simulink model "gtm_design"  (R2025b)
settings: Solver=ode2  StartTime=0.0  StopTime=1000  FixedStep=Timestep  MaxStep=0.1  MinStep=0.005  RelTol=1e-5
StopFcn:
  | MWSout=grabmws(bdroot);
  | MWSout.lastrun=datestr(now);
values from neighbouring files (symbols this model uses):
  AltMap = [0 20 40 60 80 100 120 140 160 180 200 220 ... (2938 elements, 1469x2)]    [WPs.mat]    (also in create_WPs.m = [s_alt, alt_ref])
  ApproachParams = [29.3870633886 40.9266984885 1000 29.3345096172 40.9077524395 408.9474942 29.321008 40.902885 318.9474942 244.5 2.5 90]    [WPs.mat]    (also in alternative_trajectory.mat; create_WPs.m = TRJ.ApproachParams; guidance.m = [; trajectory.mat)
  psi_deg = [0 0 0 0 0 0 0 0 0 0 0 0 ... (60 elements, 60x1)]    [WPs.mat]    (also in create_WPs.m = zeros(size(lat_wp)))
  WPs = [29.3 29.3 29.3 29.3 29.3 29.3 29.3 29.3 29.3 29.3 29.3 29.3 ... (240 elements, 60x4)]    [WPs.mat]    (also in create_WPs.m = [      lon_wp,      lat_wp,      alt_wp,      tas_kts])
undefined symbols (not defined in the file or in its folder): Aero, aftfuel, aftfuel_pos, AILL, AILLC, AILR, AILRC, alpha_deg, altitude_ft, Ax_g, Ay_g, Az_g, b, beta_deg, bias, BRAKEC, Cbar, cg_pos0, cg_shift_gear, DamageCase, DamageModels, DamageOnsetTime, ELLIB, ELLIBC, ELLOB, ELLOBC, ELRIB, ELRIBC, ELROB, ELROBC, engl_ang, engl_pos, engr_ang, engr_pos, FLAPLIB, FLAPLIC, FLAPLOB, FLAPLOC, FLAPRIB, FLAPRIC, FLAPROB, FLAPROC, FuelUsed_Init, fwdfuel, fwdfuel_pos, GEAR, GEARC, Inertia0, Inertia_shift_gear, InitialTime, Ixx_model, Iyy_model, Izz_model, KTAS, LandingGear, LengON, LinearizeModeOn, ln, NAV_altitude_m, NAV_latitude_deg ... (+62)
libraries: simulink_need_slupdate x30, simulink x11, slpidlib x7, simulink_extras x6, aerolibfltsims x2
(part 8 of 8)

== system gtm_design/Input Generator/Winds/Turbulence  Model/Dryden Model/Longitudinal Turbulence/filter parameters/Tm-4511 severe data ==
  note: "Light" and "Moderate" sigmas are ZERO below 1km alt.
      | Table 2-79 does not define them.
  "alt, m" : Inport
  intensity : Inport  Port=2
  "Longitudinal Scale, m TM-4511 Table 2-79" : Lookup  InputValues=[0 10 20 30 40 50 60 70 80 90 100 200 304.8 305 762 769 900 1000 2000 4000 6000 8000 10000 12000 14000 16000]  Table=[21 21 33 43 52 61 68 75 82 89 95 149 196 300 300 533 533 832 902 1040 1040 1040 1230 1800 2820 3400]
  "Longitudinal sigma, m/s light TM-4511 Table 2-79" : Lookup  InputValues="[10 20 30 40 50 60 70 80 90 100 200 304.8 305 400  762 769 1000 2000 4000 6000 8000 10000 12000 14000 16000]"  Table="[0   0   0   0   0   0   0   0   0    0    0    0   0   0   0   0   .17  .17  .2   .21   .22   .22   .25   .26   .24   ]"
  "Longitudinal sigma, m/s moderate TM-4511 Table 2-79" : Lookup  InputValues="[10 20 30 40 50 60 70 80 90 100 200 304.8 305 400  762 769 1000 2000 4000 6000 8000 10000 12000 14000 16000]"  Table="[0   0  0    0    0   0  0  0   0   0     0    0      0     0      0    0  1.65  1.65 2.04 2.13 2.15 2.23 2.47 2.62 2.44]"
  "Longitudinal sigma, m/s severe TM-4511 Table 2-79" : Lookup  InputValues="[10 20 30 40 50 60 70 80 90 100 200 304.8 305 400  762 769 1000 2000 4000 6000 8000 10000 12000 14000 16000]"  Table=[2.31 2.58 2.75 2.88 2.98 3.07 3.15 3.22 3.28 3.33 3.72 3.95 4.37 4.39 4.39 5.7 5.7 5.8 6.24 7.16 7.59 7.72 7.89 6.93 5]
  Multiport Switch : MultiPortSwitch
  "sigma, m/s" : Outport
  "scale length, m" : Outport  Port=2
  wires:
  "alt, m"/1 -> "Longitudinal sigma, m/s severe TM-4511 Table 2-79"/1, "Longitudinal Scale, m TM-4511 Table 2-79"/1, "Longitudinal sigma, m/s moderate TM-4511 Table 2-79"/1, "Longitudinal sigma, m/s light TM-4511 Table 2-79"/1
  "Longitudinal Scale, m TM-4511 Table 2-79"/1 -> "scale length, m"/1
  Multiport Switch/1 -> "sigma, m/s"/1
  "Longitudinal sigma, m/s severe TM-4511 Table 2-79"/1 -> Multiport Switch/4
  "Longitudinal sigma, m/s moderate TM-4511 Table 2-79"/1 -> Multiport Switch/3
  "Longitudinal sigma, m/s light TM-4511 Table 2-79"/1 -> Multiport Switch/2
  intensity/1 -> Multiport Switch/1

== system gtm_design/Input Generator/Winds/Turbulence  Model/Dryden Model/Vertical Turbulence/SubSystem/MIL-STD-1797A APPENDIX A  ==
  note: This data from Fig 262, pg 652
  "alt, m" : Inport
  intensity : Inport  Port=2
  "0.1*mean wind, fps sigma w = to 2.5f/s * intensity Fig 263, pg 654" : Gain  Gain=2.5  SaturateOnIntegerOverflow=on  OutDataTypeStr=Inherit: Same as input  ParamDataTypeStr=Inherit: Same as input
  1 : Constant  Value=500
  2 : Constant  Value=.15
  Demux : Demux  Outputs=2
      settings: DisplayOption=none
  "L w = min(500, alt/2)" : Fcn  Expr=u(1)/2
  "Light sigma, f/s" : Lookup  InputValues=[2000 9000 18000 100000]  Table=[5 5 3 3]
  MinMax : MinMax  Inputs=2  InputSameDT=on  SaturateOnIntegerOverflow=on
  MinMax1 : MinMax  Function=max  Inputs=2  InputSameDT=on  SaturateOnIntegerOverflow=on
  Multiport Switch : MultiPortSwitch
  Mux : Mux  Inputs=2
  Mux1 : Mux  Inputs=2
  Product : Product  InputSameDT=on  SaturateOnIntegerOverflow=on  OutDataTypeStr=Inherit: Same as first input
  "Scale Length, ft" : Constant  Value=1750/2
  Ux / U20 : Fcn  Expr=ln(u(1)/.15)/ln(20/.15)
  alt >2000 ft : Switch  Threshold=2000
  "ft -> m" : Gain  Gain=.3048  SaturateOnIntegerOverflow=on  OutDataTypeStr=Inherit: Same as input  ParamDataTypeStr=Inherit: Same as input
  "m -> ft" : Gain  Gain=1/.3048  SaturateOnIntegerOverflow=on  OutDataTypeStr=Inherit: Same as input  ParamDataTypeStr=Inherit: Same as input
  "moderate sigma, f/s" : Lookup  InputValues=[2000 12000 44000 100000]  Table=[10 10 3 3]
  "severe sigma, f/s" : Lookup  InputValues=[2000 5000 22000 80000 100000]  Table=[15.5 21.5 21.5 3 3]
  "sigma, m/s" : Outport
  "scale length, m" : Outport  Port=2
  wires:
  "Light sigma, f/s"/1 -> Multiport Switch/2
  "moderate sigma, f/s"/1 -> Multiport Switch/3
  "severe sigma, f/s"/1 -> Multiport Switch/4
  "alt, m"/1 -> "m -> ft"/1
  Multiport Switch/1 -> Mux/1
  Mux/1 -> alt >2000 ft/1
  intensity/1 -> Multiport Switch/1, "0.1*mean wind, fps sigma w = to 2.5f/s * intensity Fig 263, pg 654"/1
  "Scale Length, ft"/1 -> Mux/2
  "m -> ft"/1 -> alt >2000 ft/2, "severe sigma, f/s"/1, "Light sigma, f/s"/1, "moderate sigma, f/s"/1, "L w = min(500, alt/2)"/1, MinMax1/2
  Mux1/1 -> alt >2000 ft/3
  Demux/2 -> "scale length, m"/1
  Demux/1 -> "sigma, m/s"/1
  alt >2000 ft/1 -> "ft -> m"/1
  "ft -> m"/1 -> Demux/1
  1/1 -> MinMax/1
  "L w = min(500, alt/2)"/1 -> MinMax/2
  2/1 -> MinMax1/1
  MinMax1/1 -> Ux / U20/1
  Ux / U20/1 -> Product/2
  "0.1*mean wind, fps sigma w = to 2.5f/s * intensity Fig 263, pg 654"/1 -> Product/1
  Product/1 -> Mux1/1
  MinMax/1 -> Mux1/2

== system gtm_design/Input Generator/Winds/Turbulence  Model/Dryden Model/Vertical Turbulence/SubSystem/Tm-4511 severe data ==
  note: "Light" and "Moderate" sigmas are ZERO below 1km alt.
      | Table 2-79 does not define them.
  "alt, m" : Inport
  intensity : Inport  Port=2
  Multiport Switch : MultiPortSwitch
  "Vertical sigma, m/s light TM-4511 Table 2-79" : Lookup  InputValues="[10 20 30 40 50 60 70 80 90 100 200 304.8 305 400  762 769 1000 2000 4000 6000 8000 10000 12000 14000 16000]"  Table="[0   0   0   0   0   0   0   0   0    0    0    0   0   0   0   0   .14  .14  .17   .17   .17   .17   .18   .19   .21   ]"
  "Vertical sigma, m/s moderate TM-4511 Table 2-79" : Lookup  InputValues="[10 20 30 40 50 60 70 80 90 100 200 304.8 305 400  762 769 1000 2000 4000 6000 8000 10000 12000 14000 16000]"  Table="[0   0  0    0    0   0  0  0   0   0     0    0      0     0      0    0  1.36  1.43 1.68 1.69 1.695 1.73 1.79 1.91 2.1]"
  "Vertical Scale, m TM-4511 Table 2-79" : Lookup  InputValues=[0 10 20 30 40 50 60 70 80 90 100 200 304.8 305 762 769 900 1000 2000 4000 6000 8000 10000 12000 14000 16000]  Table=[ 5 5 11 17 23 29 35 41 47 53 59 123 192 300 300 533 533 624 831 972 1010 980 1100 1540 2120 2600]
  "Vertical sigma, m/s severe TM-4511 Table 2-79" : Lookup  InputValues=[10 20 30 40 50 60 70 80 90 100 200 304.8 305 762 769 900 1000 2000 4000 6000 8000 10000 12000 14000 16000]  Table=[1.15 1.46 1.71 1.89 2.05 2.19 2.32 2.43 2.54 2.64 3.38 3.95 4.39 4.39 5.7 5.7 4.67 4.75 5.13 5.69 5.98 6 5.71 5.05 4.31]
  "sigma, m/s" : Outport
  "scale length, m" : Outport  Port=2
  wires:
  "alt, m"/1 -> "Vertical Scale, m TM-4511 Table 2-79"/1, "Vertical sigma, m/s severe TM-4511 Table 2-79"/1, "Vertical sigma, m/s moderate TM-4511 Table 2-79"/1, "Vertical sigma, m/s light TM-4511 Table 2-79"/1
  "Vertical Scale, m TM-4511 Table 2-79"/1 -> "scale length, m"/1
  Multiport Switch/1 -> "sigma, m/s"/1
  "Vertical sigma, m/s moderate TM-4511 Table 2-79"/1 -> Multiport Switch/3
  "Vertical sigma, m/s light TM-4511 Table 2-79"/1 -> Multiport Switch/2
  intensity/1 -> Multiport Switch/1
  "Vertical sigma, m/s severe TM-4511 Table 2-79"/1 -> Multiport Switch/4

== matlab function gtm_design/GTM_T2/EOM/Aircraft 6DOF/EulerDot ==
  data: pqr input size=3; deuler output size=3; euler input size=3
function deuler = e2de(pqr,euler)
% This block supports an embeddable subset of the MATLAB language.
% See the help menu for details. 

P=pqr(1);
Q=pqr(2);
R=pqr(3);

phi=euler(1);
theta=euler(2);
psi=euler(3);

c_phi=cos(phi);
s_phi=sin(phi);
c_theta=cos(theta);
s_theta=sin(theta);

phi_dot   = P + (1/c_theta)*(s_phi*s_theta*Q + c_phi*s_theta*R);
theta_dot = c_phi*Q - s_phi*R;
psi_dot   = (1/c_theta)*(s_phi*Q + c_phi*R);

deuler=[phi_dot; theta_dot; psi_dot];

== matlab function gtm_design/GTM_T2/EOM/Aircraft 6DOF/Form Inertia Matrix ==
  data: Ixx input double size=1; I output size=[3 3]; Iyy input size=1; Izz input size=1; Ixz input size=1; Iyz input size=1; Ixy input size=1; InvI output size=[3 3]
function [I,InvI] = Inertia(Ixx,Iyy,Izz,Ixz,Iyz,Ixy)
% This block supports an embeddable subset of the MATLAB language.
% See the help menu for details. 

I=[ Ixx, -Ixy, -Ixz;
   -Ixy,  Iyy, -Iyz;
   -Ixz, -Iyz,   Izz ];

det = Ixx*Iyy*Izz-Ixx*Iyz^2-Ixy^2*Izz-2*Ixy*Ixz*Iyz-Ixz^2*Iyy;

adjoint=[...
Iyy*Izz-Iyz^2,    Ixy*Izz+Ixz*Iyz, Ixy*Iyz+Ixz*Iyy;...
Ixy*Izz+Ixz*Iyz,   Ixx*Izz-Ixz^2,  Ixx*Iyz+Ixy*Ixz;...
Ixy*Iyz+Ixz*Iyy,  Ixx*Iyz+Ixy*Ixz,   Ixx*Iyy-Ixy^2     ];

InvI=adjoint/det;

== matlab function gtm_design/GTM_T2/Engines/Engine Alignment ==
  data: T output; Tl input; hl input; Tr input; hr input; TL output; engl_ang parameter; engr_ang parameter; TR output; H output
function [T,TL,TR,H] = eng_angles(Tl,hl,Tr,hr,engl_ang,engr_ang)
% This block supports an embeddable subset of the MATLAB language.
% See the help menu for details. 

% Using the engine alignment angles (set in AC_params_T2.m), compute the 
% off-axis thrust and angular momentum terms.

TL = Tl*[cosd(engl_ang(2))*cosd(engl_ang(3));...
         sind(engl_ang(3));...
         -sind(engl_ang(2))*cosd(engl_ang(3))];
TR = Tr*[cosd(engr_ang(2))*cosd(engr_ang(3));...
         sind(engr_ang(3));...
         -sind(engr_ang(2))*cosd(engr_ang(3))];  
T = TL+TR;

H = hl*[cosd(engl_ang(2))*cosd(engl_ang(3));...
         sind(engl_ang(3));...
         -sind(engl_ang(2))*cosd(engl_ang(3))] + ...
         hr*[cosd(engr_ang(2))*cosd(engr_ang(3));...
         sind(engr_ang(3));...
         -sind(engr_ang(2))*cosd(engr_ang(3))];

== matlab function gtm_design/GTM_T2/Engines/Left_Engine Jetcat P70/Simple Ram Drag Model ==
  data: ram_drag output; qbar input; S input; ram_drag_coef parameter
function ram_drag =   ram_drag(qbar,S,ram_drag_coef)
% This block supports the Embedded MATLAB subset.
% See the help menu for details. 

ram_drag = ram_drag_coef.*qbar.*S;
return

== matlab function gtm_design/GTM_T2/Engines/Right_Engine Jetcat P70/Simple Ram Drag Model ==
  data: ram_drag output; qbar input; S input; ram_drag_coef parameter
function ram_drag =   ram_drag(qbar,S,ram_drag_coef)
% This block supports the Embedded MATLAB subset.
% See the help menu for details. 

ram_drag = ram_drag_coef.*qbar.*S;
return

== matlab function gtm_design/Input Generator/FCS/Waypoint Tracking ==
  settings: updateMethod=DISCRETE  sampleTime=0.01
  data: lon_deg input; h_ref output; lat_deg input; alt_ft input; psi_deg input; TAS_kts input; beta_deg input; WPs input; AltMap input; ApproachParams input; Ts input; reset input; psi_ref output; TAS_ref output; beta_ref output; wp_idx output; status output; e_ct output; dist_to_wp output; along_m output
function [h_ref, psi_ref, TAS_ref, beta_ref, wp_idx, status, e_ct, dist_to_wp, along_m] = ...
    WP_Tracker(lon_deg, lat_deg, alt_ft, psi_deg, TAS_kts, beta_deg, WPs, AltMap, ApproachParams, Ts, reset)
%#codegen
%
% WPs format:
%   WPs(:,1) = lon_deg
%   WPs(:,2) = lat_deg
%   WPs(:,3) = alt_ft
%   WPs(:,4) = TAS_kts
%
% AltMap format:
%   AltMap(:,1) = station_m
%   AltMap(:,2) = alt_ref_ft
%
% ApproachParams format:
%   1  = FAF_lon_deg
%   2  = FAF_lat_deg
%   3  = FAF_alt_ft
%   4  = FLARE_lon_deg
%   5  = FLARE_lat_deg
%   6  = FLARE_alt_ft
%   7  = TD_lon_deg
%   8  = TD_lat_deg
%   9  = TD_alt_ft
%   10 = runway_heading_deg
%   11 = glide_angle_deg
%   12 = flare_alt_agl_ft

%% ============================================================
% USER PARAMETERS
% =============================================================

lat0_deg = 40.88;
lon0_deg = 29.30;

% Normal WP acceptance
R_accept_m = 80.0;

% Turn WP acceptance
% Dönüş waypointlerinde daha erken segment değişimi için kullanılır.
% 220-300 m arası denenebilir.
R_accept_turn_m = 320.0;

% Bir WP'nin dönüş WP'si sayılması için minimum rota değişimi
turn_angle_min_deg = 25.0;

R_final_m = 50.0;

lookahead_time_s = 4.0;
Ld_min_m = 80.0;
Ld_max_m = 450.0;

psi_exp_small_err_deg = 25.0;
psi_exp_large_err_deg = 65.0;

chi_corr_lim_deg = 30.0;

exp_Ld_factor = 1.5;
exp_Ld_min_m  = 150.0;
exp_Ld_max_m  = 800.0;

psi_rate_lim_degps = 20.0;
h_rate_lim_ftps    = 25.0;
TAS_rate_lim_ktsps = 5.0;

TAS_min_kts = 0.0;
TAS_max_kts = 120.0;

% Normal AltMap station protection
alt_back_window_m = 30.0;
alt_fwd_window_min_m = 150.0;
alt_fwd_window_time_s = 5.0;
alt_station_rate_gain = 1.10;

% Approach geometry activation gates
approach_pre_faf_margin_m = 1500.0;
approach_xtrack_gate_m    = 1200.0;
approach_after_td_m       = 500.0;

% Smooth vertical curve at FAF
faf_vertical_curve_m = 600.0;

%% ============================================================
% PERSISTENT STATES
% =============================================================

persistent targetIdx initialized ...
           startN startE startAlt startTAS ...
           hLast psiLast TASLast ...
           sAltLast

if isempty(initialized) || reset > 0.5

    targetIdx = int32(1);

    [startN, startE] = ll2ne_simple(lat_deg, lon_deg, lat0_deg, lon0_deg);

    startAlt = alt_ft;
    startTAS = TAS_kts;

    hLast   = alt_ft;
    psiLast = wrap180(psi_deg);
    TASLast = TAS_kts;

    sAltLast = 0.0;

    initialized = true;

end

Ts_eff = max(Ts, 1.0e-6);

Nwp = int32(size(WPs, 1));

%% ============================================================
% EMPTY / INVALID MISSION PROTECTION
% =============================================================

if Nwp < int32(1)

    h_ref      = alt_ft;
    psi_ref    = wrap180(psi_deg);
    TAS_ref    = TAS_kts;
    beta_ref   = 0.0;
    wp_idx     = 0.0;
    status     = -1.0;
    e_ct       = 0.0;
    dist_to_wp = 0.0;
    along_m    = 0.0;

    return;

end

if targetIdx < int32(1)
    targetIdx = int32(1);
end

if targetIdx > Nwp
    targetIdx = Nwp;
end

%% ============================================================
% CURRENT AIRCRAFT POSITION IN LOCAL NORTH-EAST FRAME
% =============================================================

[pN, pE] = ll2ne_simple(lat_deg, lon_deg, lat0_deg, lon0_deg);

%% ============================================================
% ADVANCE WAYPOINT IF NEEDED
% =============================================================

for iter = 1:200

    if iter > double(Nwp)
        break;
    end

    [AN, AE, ~, ~] = getSegmentStart(targetIdx, WPs, ...
        startN, startE, startAlt, startTAS, lat0_deg, lon0_deg);

    [BN, BE, ~, ~] = getWaypoint(targetIdx, WPs, lat0_deg, lon0_deg);

    dN = BN - AN;
    dE = BE - AE;

    L = sqrt(dN*dN + dE*dE);

    if L < 1.0

        qN = cosd(psiLast);
        qE = sind(psiLast);
        s  = 0.0;

    else

        qN = dN / L;
        qE = dE / L;
        s  = (pN - AN)*qN + (pE - AE)*qE;

    end

    dToB_N = pN - BN;
    dToB_E = pE - BE;
    distB  = sqrt(dToB_N*dToB_N + dToB_E*dToB_E);

    e_ct_switch = -qE*(pN - AN) + qN*(pE - AE);

    % ------------------------------------------------------------
    % Turn-aware waypoint acceptance radius
    % ------------------------------------------------------------
    % Düz WP'lerde normal radius kullanılır.
    % Dönüş WP'lerinde daha büyük radius kullanılır.
    %
    % Bu sayede tracker dönüş WP'sine çok geç kalmadan bir sonraki
    % segmente geçer ve psi_ref köşeli kırılmak yerine daha erken
    % dönmeye başlar.

    isTurnWP = isTurningWaypoint(targetIdx, WPs, startN, startE, ...
        lat0_deg, lon0_deg, turn_angle_min_deg);

    if isTurnWP
        R_accept_eff = R_accept_turn_m;
    else
        R_accept_eff = R_accept_m;
    end

    passed_halfplane = (s >= L);
    near_wp = (distB <= R_accept_eff);
    near_path_lateral = (abs(e_ct_switch) <= R_accept_eff);

    if targetIdx < Nwp && (near_wp || (passed_halfplane && near_path_lateral) || L < 1.0)
        targetIdx = targetIdx + int32(1);
    else
        break;
    end

end

%% ============================================================
% ACTIVE SEGMENT GEOMETRY
% =============================================================

[AN, AE, Aalt, ATAS] = getSegmentStart(targetIdx, WPs, ...
    startN, startE, startAlt, startTAS, lat0_deg, lon0_deg);

[BN, BE, Balt, BTAS] = getWaypoint(targetIdx, WPs, lat0_deg, lon0_deg);

dN = BN - AN;
dE = BE - AE;

L = sqrt(dN*dN + dE*dE);

if L < 1.0

    qN = cosd(psiLast);
    qE = sind(psiLast);
    s  = 0.0;

else

    qN = dN / L;
    qE = dE / L;
    s  = (pN - AN)*qN + (pE - AE)*qE;

end

s_clamped = sat(s, 0.0, max(L, 1.0));

e_ct = -qE*(pN - AN) + qN*(pE - AE);

dToB_N = pN - BN;
dToB_E = pE - BE;
dist_to_wp = sqrt(dToB_N*dToB_N + dToB_E*dToB_E);

along_m = s;

%% ============================================================
% LOOKAHEAD / CARROT POINT
% =============================================================

TAS_ms = max(TAS_kts, 1.0) * 0.514444;

Ld = lookahead_time_s * TAS_ms;
Ld = sat(Ld, Ld_min_m, Ld_max_m);

if L < 1.0
    s_LA = 0.0;
else
    s_LA = sat(s_clamped + Ld, 0.0, L);
end

alpha_LA = 1.0;

if L >= 1.0
    alpha_LA = sat(s_LA / L, 0.0, 1.0);
end

N_LA = AN + alpha_LA*dN;
E_LA = AE + alpha_LA*dE;

dLA_N = N_LA - pN;
dLA_E = E_LA - pE;

dist_LA = sqrt(dLA_N*dLA_N + dLA_E*dLA_E);

if dist_LA < 1.0
    psi_carrot = psiLast;
else
    psi_carrot = atan2d(dLA_E, dLA_N);
end

psi_carrot = wrap180(psi_carrot);

%% ============================================================
% HYBRID PSI REFERENCE GENERATION
% =============================================================

psi_carrot_raw = psi_carrot;

if L < 1.0
    chi_path = psiLast;
else
    chi_path = atan2d(qE, qN);
end

chi_path = wrap180(chi_path);

Ld_exp = exp_Ld_factor * Ld;
Ld_exp = sat(Ld_exp, exp_Ld_min_m, exp_Ld_max_m);

chi_corr = atan2d(-e_ct, Ld_exp);
chi_corr = sat(chi_corr, -chi_corr_lim_deg, chi_corr_lim_deg);

psi_exp_raw = wrap180(chi_path + chi_corr);

err_heading_path   = abs(wrap180(chi_path       - psi_deg));
err_heading_carrot = abs(wrap180(psi_carrot_raw - psi_deg));

heading_err_for_mode = min(err_heading_path, err_heading_carrot);

blend_den = max(psi_exp_large_err_deg - psi_exp_small_err_deg, 1.0);

mu_carrot = (heading_err_for_mode - psi_exp_small_err_deg) / blend_den;
mu_carrot = smoothstep01(mu_carrot);

psi_raw = angleLerpDeg(psi_exp_raw, psi_carrot_raw, mu_carrot);

if heading_err_for_mode < psi_exp_small_err_deg
    psi_raw = psi_exp_raw;
end

psi_raw = wrap180(psi_raw);

%% ============================================================
% ALTITUDE AND TAS REFERENCES
% =============================================================

% ------------------------------------------------------------
% 1) Normal altitude from AltMap
% ------------------------------------------------------------

alt_fwd_window_m = max(alt_fwd_window_min_m, TAS_ms * alt_fwd_window_time_s);

s_alt_candidate = getMissionStationClosestWindowed( ...
    pN, pE, WPs, startN, startE, lat0_deg, lon0_deg, ...
    sAltLast, alt_back_window_m, alt_fwd_window_m);

if s_alt_candidate < sAltLast
    s_alt_candidate = sAltLast;
end

sAlt_rate_max = max(TAS_ms, 1.0) * alt_station_rate_gain;
sAlt_step_max = sAlt_rate_max * Ts_eff;

if s_alt_candidate > sAltLast + sAlt_step_max
    s_alt = sAltLast + sAlt_step_max;
else
    s_alt = s_alt_candidate;
end

sAltLast = s_alt;

h_fallback = Aalt + alpha_LA*(Balt - Aalt);
h_altmap = getAltFromMap(s_alt, AltMap, h_fallback);

% ------------------------------------------------------------
% 2) Approach altitude protection / override
% ------------------------------------------------------------
%
% appMode:
%   0 = not in approach geometry, use AltMap
%   1 = before FAF, do not allow h_ref below FAF altitude
%   2 = FAF -> FLARE, use glide slope geometry
%   3 = FLARE -> TOUCHDOWN, use flare arc geometry
%   4 = after touchdown, hold touchdown altitude

[h_app, appMode] = getApproachAltitudeRef( ...
    pN, pE, ApproachParams, lat0_deg, lon0_deg, ...
    approach_pre_faf_margin_m, approach_xtrack_gate_m, approach_after_td_m, ...
    faf_vertical_curve_m);

[faf_alt_floor, before_faf] = getFafAltitudeFloor( ...
    pN, pE, ApproachParams, lat0_deg, lon0_deg);

if appMode == int32(0)

    h_raw = h_altmap;

    if before_faf
        h_raw = max(h_raw, faf_alt_floor);
    end

elseif appMode == int32(1)

    h_raw = max(h_altmap, h_app);

else

    h_raw = h_app;

end

% ------------------------------------------------------------
% 3) TAS reference
% ------------------------------------------------------------
%
% TAS için alpha_LA kullanılmaz.
% alpha_LA carrot/lookahead guidance içindir.
% TAS gerçek segment ilerlemesi s/L ile hesaplanır.

if L < 1.0
    alpha_TAS = 1.0;
else
    alpha_TAS = sat(s / L, 0.0, 1.0);
end

TAS_raw = ATAS + alpha_TAS*(BTAS - ATAS);
TAS_raw = sat(TAS_raw, TAS_min_kts, TAS_max_kts);

%% ============================================================
% FINAL WAYPOINT LOGIC
% =============================================================

status = 1.0;

if targetIdx == Nwp && dist_to_wp <= R_final_m

    status  = 2.0;

    % Do NOT force h_raw to final waypoint altitude here.
    TAS_raw = BTAS;
    psi_raw = psiLast;

end

%% ============================================================
% RATE LIMIT REFERENCES
% =============================================================

h_ref = rateLimitScalar(hLast, h_raw, h_rate_lim_ftps, Ts_eff);
hLast = h_ref;

TAS_ref = rateLimitScalar(TASLast, TAS_raw, TAS_rate_lim_ktsps, Ts_eff);
TAS_ref = sat(TAS_ref, TAS_min_kts, TAS_max_kts);
TASLast = TAS_ref;

psi_ref = rateLimitAngleDeg(psiLast, psi_raw, psi_rate_lim_degps, Ts_eff);
psi_ref = wrap180(psi_ref);
psiLast = psi_ref;

%% ============================================================
% SIDESLIP REFERENCE
% =============================================================

beta_ref = 0.0;

% beta_deg is kept in the function input only to preserve the Simulink port.
unused_beta = beta_deg; %#ok<NASGU>

wp_idx = double(targetIdx);

end

%% ============================================================
% LOCAL FUNCTIONS
% =============================================================

function [N, E] = ll2ne_simple(lat_deg, lon_deg, lat0_deg, lon0_deg)

R_E = 6378137.0;

dLat = deg2rad_local(lat_deg - lat0_deg);
dLon = deg2rad_local(lon_deg - lon0_deg);

lat0_rad = deg2rad_local(lat0_deg);

N = R_E * dLat;
E = R_E * cos(lat0_rad) * dLon;

end

function [N, E, alt_ft, TAS_kts] = getWaypoint(idx, WPs, lat0_deg, lon0_deg)

k = double(idx);

lon = WPs(k, 1);
lat = WPs(k, 2);

[N, E] = ll2ne_simple(lat, lon, lat0_deg, lon0_deg);

alt_ft  = WPs(k, 3);
TAS_kts = WPs(k, 4);

end

function [N, E, alt_ft, TAS_kts] = getSegmentStart(idx, WPs, ...
    startN, startE, startAlt, startTAS, lat0_deg, lon0_deg)

if idx <= int32(1)

    N       = startN;
    E       = startE;
    alt_ft  = startAlt;
    TAS_kts = startTAS;

else

    prevIdx = idx - int32(1);
    [N, E, alt_ft, TAS_kts] = getWaypoint(prevIdx, WPs, lat0_deg, lon0_deg);

end

end

function isTurn = isTurningWaypoint(idx, WPs, startN, startE, ...
    lat0_deg, lon0_deg, turnAngleMinDeg)

isTurn = false;

Nwp = int32(size(WPs, 1));

% Son WP için dönüş kontrolü yapılmaz.
if idx >= Nwp
    return;
end

% Current waypoint B.
[BN, BE, ~, ~] = getWaypoint(idx, WPs, lat0_deg, lon0_deg);

% Previous point A.
if idx <= int32(1)
    AN = startN;
    AE = startE;
else
    [AN, AE, ~, ~] = getWaypoint(idx - int32(1), WPs, lat0_deg, lon0_deg);
end

% Next waypoint C.
[CN, CE, ~, ~] = getWaypoint(idx + int32(1), WPs, lat0_deg, lon0_deg);

v1N = BN - AN;
v1E = BE - AE;

v2N = CN - BN;
v2E = CE - BE;

L1 = sqrt(v1N*v1N + v1E*v1E);
L2 = sqrt(v2N*v2N + v2E*v2E);

if L1 < 1.0 || L2 < 1.0
    return;
end

q1N = v1N / L1;
q1E = v1E / L1;

q2N = v2N / L2;
q2E = v2E / L2;

dot12 = q1N*q2N + q1E*q2E;
dot12 = sat(dot12, -1.0, 1.0);

turnAngleDeg = acosd(dot12);

isTurn = turnAngleDeg >= turnAngleMinDeg;

end

function sBest = getMissionStationClosestWindowed( ...
    pN, pE, WPs, startN, startE, lat0_deg, lon0_deg, ...
    sCenter, backWindow, fwdWindow)

Nwp = int32(size(WPs, 1));

sWindowStart = sCenter - backWindow;
sWindowEnd   = sCenter + fwdWindow;

if sWindowStart < 0.0
    sWindowStart = 0.0;
end

sCum = 0.0;
sBest = sCenter;
bestDist2 = 1.0e30;
found = false;

prevN = startN;
prevE = startE;

for k = int32(1):Nwp

    [currN, currE, ~, ~] = getWaypoint(k, WPs, lat0_deg, lon0_deg);

    dN = currN - prevN;
    dE = currE - prevE;

    Lseg = sqrt(dN*dN + dE*dE);

    if Lseg > 1.0

        segStart = sCum;
        segEnd   = sCum + Lseg;

        overlapStart = max(segStart, sWindowStart);
        overlapEnd   = min(segEnd,   sWindowEnd);

        if overlapEnd >= overlapStart

            qN = dN / Lseg;
            qE = dE / Lseg;

            sLocal = (pN - prevN)*qN + (pE - prevE)*qE;
            sLocal = sat(sLocal, 0.0, Lseg);

            sCandidate = sCum + sLocal;
            sCandidate = sat(sCandidate, overlapStart, overlapEnd);

            sLocalCandidate = sCandidate - sCum;

            projN = prevN + sLocalCandidate*qN;
            projE = prevE + sLocalCandidate*qE;

            errN = pN - projN;
            errE = pE - projE;

            dist2 = errN*errN + errE*errE;

            if dist2 < bestDist2
                bestDist2 = dist2;
                sBest = sCandidate;
                found = true;
            end

        end

        sCum = sCum + Lseg;

    end

    prevN = currN;
    prevE = currE;

end

if ~found
    sBest = sCenter;
end

end

function h = getAltFromMap(sQuery, AltMap, fallback_h)

M = int32(size(AltMap, 1));
C = int32(size(AltMap, 2));

if M < int32(1) || C < int32(2)
    h = fallback_h;
    return;
end

if M == int32(1)
    h = AltMap(1, 2);
    return;
end

sFirst = AltMap(1, 1);
hFirst = AltMap(1, 2);

sLast = AltMap(double(M), 1);
hLastMap = AltMap(double(M), 2);

if sQuery <= sFirst
    h = hFirst;
    return;
end

if sQuery >= sLast
    h = hLastMap;
    return;
end

h = fallback_h;

for kk = 1:double(M - int32(1))

    s0 = AltMap(kk, 1);
    s1 = AltMap(kk+1, 1);

    h0 = AltMap(kk, 2);
    h1 = AltMap(kk+1, 2);

    if s1 > s0

        if sQuery >= s0 && sQuery <= s1

            alpha = (sQuery - s0) / (s1 - s0);
            alpha = sat(alpha, 0.0, 1.0);

            h = h0 + alpha*(h1 - h0);
            return;

        end

    end

end

end

function [h_app, appMode] = getApproachAltitudeRef( ...
    pN, pE, ApproachParams, lat0_deg, lon0_deg, ...
    preFafMargin_m, xtrackGate_m, afterTd_m, fafVerticalCurve_m)

h_app = 0.0;
appMode = int32(0);

if numel(ApproachParams) < 12
    return;
end

faf_lon   = ApproachParams(1);
faf_lat   = ApproachParams(2);
faf_alt   = ApproachParams(3);

flare_lon = ApproachParams(4);
flare_lat = ApproachParams(5);
flare_alt = ApproachParams(6);

td_lon    = ApproachParams(7);
td_lat    = ApproachParams(8);
td_alt    = ApproachParams(9);

rwy_hdg   = ApproachParams(10);
glide_deg = abs(ApproachParams(11));
flare_agl_ft = max(ApproachParams(12), 0.0);

if glide_deg < 0.1
    glide_deg = 0.1;
end

[fafN, fafE] = ll2ne_simple(faf_lat, faf_lon, lat0_deg, lon0_deg);
[flareN, flareE] = ll2ne_simple(flare_lat, flare_lon, lat0_deg, lon0_deg);
[tdN, tdE] = ll2ne_simple(td_lat, td_lon, lat0_deg, lon0_deg);

qN = cosd(rwy_hdg);
qE = sind(rwy_hdg);

% Positive distance means aircraft is before touchdown on final direction.
d_to_td = (tdN - pN)*qN + (tdE - pE)*qE;

d_faf_to_td   = (tdN - fafN)*qN + (tdE - fafE)*qE;
d_flare_to_td = (tdN - flareN)*qN + (tdE - flareE)*qE;

if d_faf_to_td < d_flare_to_td

    tmp = d_faf_to_td;
    d_faf_to_td = d_flare_to_td;
    d_flare_to_td = tmp;

end

if d_flare_to_td < 0.0
    d_flare_to_td = 0.0;
end

rN = pN - tdN;
rE = pE - tdE;

xtrack = -qE*rN + qN*rE;

% Only protect/override altitude near extended final corridor.
insideCorridor = abs(xtrack) <= xtrackGate_m;
insideAlong = (d_to_td <= d_faf_to_td + preFafMargin_m) && ...
              (d_to_td >= -afterTd_m);

if ~(insideCorridor && insideAlong)
    return;
end

if d_to_td > d_faf_to_td

    % Before FAF.
    h_app = faf_alt;
    appMode = int32(1);
    return;

end

if d_to_td > d_flare_to_td

    % FAF -> FLARE.
    glide_len_m = max(d_faf_to_td - d_flare_to_td, 1.0);

    x_after_faf = d_faf_to_td - d_to_td;
    x_after_faf = sat(x_after_faf, 0.0, glide_len_m);

    % Nominal linear glide slope between FAF and FLARE.
    slope_ft_per_m = (faf_alt - flare_alt) / glide_len_m;

    % Vertical curve length.
    Lvc = fafVerticalCurve_m;
    Lvc = sat(Lvc, 1.0, 0.45*glide_len_m);

    if x_after_faf <= Lvc

        % Cubic Hermite vertical curve:
        %
        % h(0)  = FAF altitude
        % h'(0) = 0
        % h(L)  = nominal glide altitude at L
        % h'(L) = nominal glide slope

        x = x_after_faf;
        S = slope_ft_per_m;
        L = Lvc;

        drop_ft = 2.0*S*(x*x)/L - S*(x*x*x)/(L*L);

        h_app = faf_alt - drop_ft;

    else

        h_app = faf_alt - slope_ft_per_m*x_after_faf;

    end

    if h_app > faf_alt
        h_app = faf_alt;
    end

    if h_app < flare_alt
        h_app = flare_alt;
    end

    appMode = int32(2);
    return;

end

if d_to_td > 0.0

    % FLARE -> TOUCHDOWN.
    h_app = flareArcAltitudeFromDistance(d_to_td, td_alt, glide_deg, flare_agl_ft, flare_alt);
    appMode = int32(3);
    return;

end

% After touchdown.
h_app = td_alt;
appMode = int32(4);

end

function h = flareArcAltitudeFromDistance(d_to_td_m, td_alt_ft, glide_deg, flare_agl_ft, flare_alt_ft)

if d_to_td_m <= 0.0
    h = td_alt_ft;
    return;
end

gamma = deg2rad_local(glide_deg);

if flare_agl_ft <= 1.0
    h = td_alt_ft + d_to_td_m * tan(gamma) * 3.28084;
    return;
end

flare_h_m = flare_agl_ft * 0.3048;
denom = 1.0 - cos(gamma);

if denom < 1.0e-6
    h = td_alt_ft + d_to_td_m * tan(gamma) * 3.28084;
    return;
end

Rf = flare_h_m / denom;

ratio = d_to_td_m / Rf;
ratio = sat(ratio, 0.0, sin(gamma));

theta = asin(ratio);

h_agl_m = Rf * (1.0 - cos(theta));
h = td_alt_ft + h_agl_m * 3.28084;

if h > flare_alt_ft
    h = flare_alt_ft;
end

if h < td_alt_ft
    h = td_alt_ft;
end

end

function [faf_alt, before_faf] = getFafAltitudeFloor( ...
    pN, pE, ApproachParams, lat0_deg, lon0_deg)

faf_alt = 0.0;
before_faf = false;

if numel(ApproachParams) < 12
    return;
end

faf_lon = ApproachParams(1);
faf_lat = ApproachParams(2);
faf_alt = ApproachParams(3);

td_lon  = ApproachParams(7);
td_lat  = ApproachParams(8);

rwy_hdg = ApproachParams(10);

[fafN, fafE] = ll2ne_simple(faf_lat, faf_lon, lat0_deg, lon0_deg);
[tdN,  tdE ] = ll2ne_simple(td_lat,  td_lon,  lat0_deg, lon0_deg);

qN = cosd(rwy_hdg);
qE = sind(rwy_hdg);

% Positive means aircraft is before touchdown along runway heading.
d_to_td = (tdN - pN)*qN + (tdE - pE)*qE;

% FAF distance to touchdown along runway heading.
d_faf_to_td = (tdN - fafN)*qN + (tdE - fafE)*qE;

% Before FAF means still farther from touchdown than FAF is.
before_faf = d_to_td > d_faf_to_td;

end

function y = sat(x, xmin, xmax)

y = min(max(x, xmin), xmax);

end

function y = rateLimitScalar(yPrev, yCmd, rateLim, Ts)

dyMax = rateLim * Ts;

dy = yCmd - yPrev;
dy = sat(dy, -dyMax, dyMax);

y = yPrev + dy;

end

function y = rateLimitAngleDeg(yPrev, yCmd, rateLimDegps, Ts)

dyMax = rateLimDegps * Ts;

err = wrap180(yCmd - yPrev);
err = sat(err, -dyMax, dyMax);

y = wrap180(yPrev + err);

end

function a = wrap180(a)

a = mod(a + 180.0, 360.0) - 180.0;

end

function r = deg2rad_local(d)

r = d * pi / 180.0;

end

function y = smoothstep01(x)

x = sat(x, 0.0, 1.0);
y = x*x*(3.0 - 2.0*x);

end

function y = angleLerpDeg(a0, a1, mu)

mu = sat(mu, 0.0, 1.0);

da = wrap180(a1 - a0);
y = wrap180(a0 + mu*da);

end

== matlab function gtm_design/Input Generator/FCS/MATLAB Function1 ==
  data: psi_ref_deg input; e_psi output; psi_deg input
function e_psi = heading_error_deg(psi_ref_deg, psi_deg)
%#codegen
%
% Computes circular heading error.
%
% Inputs can be either:
%   -180/+180
%   or
%   0/360
%
% Output:
%   e_psi in [-180, +180]
%
% Sign convention:
%   e_psi > 0 means desired heading is clockwise/right of current heading.

dpsi = psi_ref_deg - psi_deg;

e_psi = mod(dpsi + 180.0, 360.0) - 180.0;

end

== matlab function gtm_design/GTM_T2/A/C parameters/Inertia/Mass/CG Shift/FuelBurnEffects/Polyval1/Embedded MATLAB Function ==
  data: u input; y output; p parameter
function y = fcn(u,p)
% This block supports the Embedded MATLAB subset.
% See the help menu for details. 


y = sum(p.*u.^(length(p)-1:-1:0));

== matlab function gtm_design/GTM_T2/A/C parameters/Inertia/Mass/CG Shift/fuel cg shift, cg_pos0 ==
  data: fuel_used input; y output; aftfuel parameter; fwdfuel parameter; aftfuel_pos parameter; fwdfuel_pos parameter; w0 parameter; cg_pos0 parameter
function y = fcn(fuel_used,aftfuel,fwdfuel,aftfuel_pos,fwdfuel_pos,w0,cg_pos0)
% This block supports an embeddable subset of the MATLAB language.
% See the help menu for details. 

y = w0.*cg_pos0 - min(aftfuel,fuel_used).*aftfuel_pos - max(0,fuel_used-fwdfuel).*fwdfuel_pos;

== matlab function gtm_design/GTM_T2/A/C parameters/Inertia/Mass/CG Shift/FuelBurnEffects/Polyval2/Embedded MATLAB Function ==
  data: u input; y output; p parameter
function y = fcn(u,p)
% This block supports the Embedded MATLAB subset.
% See the help menu for details. 


y = sum(p.*u.^(length(p)-1:-1:0));

== matlab function gtm_design/GTM_T2/Aero/Control Surfaces/Implement Damage Models/Implement Damage Models ==
  data: SurfVec input; DamageCase input; dC6 output; SurfGain parameter
function dC6 = fcn(SurfVec,DamageCase,SurfGain)
% This block supports an embeddable subset of the MATLAB language.
% See the help menu for details. 
damagecase = cast(round(DamageCase),'uint32');
Nsurfs=18;
if (damagecase==0),
    dC6=ones(1,Nsurfs)*(reshape(SurfVec,6,Nsurfs)');
else
  gain=squeeze(SurfGain(damagecase,:,:));
  dC6=ones(1,Nsurfs)*( transpose(reshape(SurfVec,6,Nsurfs)).*gain);
end

== matlab function gtm_design/GTM_T2/Aero/Dynamic Derviatives/Rotary Blended UnDamaged Case/Blending Function ==
  data: alpha input; omega output; beta input; tas input; pqr input; pqr_osc output; B input; Cbar input
function[omega,pqr_osc]= hykal(alpha,beta,tas,pqr,B,Cbar)
% Hybrid Kalviste blending method for use in embedded block in Simulink.
%
% Austin Murch
% Austin.M.Murch@nasa.gov

% Dimension vector outputs.
pqr_osc=zeros(3,1);
 

% Constants
dtr=pi/180;
knots2ft=1.689;

% Setup variables
pb=pqr(1);
qb=pqr(2);
rb=pqr(3);

alpha = alpha*dtr;
beta = beta*dtr;
omega = 0;

%----Hybrid Kalviste Method----%
whichcase = 0;

%Test for case 1: p_osc = 0
if cos(alpha)*cos(beta) == 0
elseif pb == 0
else
    omega = pb/(cos(alpha)*cos(beta));
    r_osc = rb - omega*sin(alpha)*cos(beta);
    if abs(r_osc) > abs(rb)
    elseif r_osc*rb < 0
    else
        whichcase = 1;
    end
end

%Test for case 2: r_osc = 0
if sin(alpha)*cos(beta) == 0
elseif rb == 0
else
    omega = rb/(sin(alpha)*cos(beta));
    p_osc = pb - omega*cos(alpha)*cos(beta);
    if abs(p_osc) > abs(pb)
    elseif p_osc*pb < 0
    else
        whichcase = 2;
    end
end

%Test for case 3: Omega = 0
if whichcase == 0
    whichcase = 3;
end

 

switch whichcase
    case 1
        omega = pb/(cos(alpha)*cos(beta));
        pqr_osc(1) = 0;        
        pqr_osc(2) = qb - omega*sin(beta);        
        pqr_osc(3) = rb - omega*sin(alpha)*cos(beta);

    case 2
        omega = rb/(sin(alpha)*cos(beta));
        pqr_osc(1) = pb - omega*cos(alpha)*cos(beta);
        pqr_osc(2) = qb - omega*sin(beta);
        pqr_osc(3) = 0;

    case 3
        pqr_osc(1) = pb;
        pqr_osc(2) = qb;
        pqr_osc(3) = rb;
        omega = 0;
end

%-----------------------------------------------% End Hybrid Kalviste

% Scale values for table lookup
b2vt=B/(2*tas*knots2ft);
c2vt=Cbar/(2*tas*knots2ft);
omega=omega*b2vt;
pqr_osc=pqr_osc.*[b2vt;c2vt;b2vt];

== matlab function gtm_design/GTM_T2/A//C parameters/Inertia//Mass//CG Shift/FuelBurnEffects/Polyval/Embedded MATLAB Function ==
  data: u input; y output; p parameter
function y = fcn(u,p)
% This block supports the Embedded MATLAB subset.
% See the help menu for details. 


y = sum(p.*u.^(length(p)-1:-1:0));

== matlab function gtm_design/GTM_T2/AuxiliaryVariables/Atmos76/atmos76 ==
  data: z input; y output; dt input
function y = layer1atm(z,dt)
% Author: Kevin Cunningham          April 20, 1992    
% Modified: Dave Cox                Aug, 14, 2008

y=zeros(6,1);

%dt=0;  % Standard Temp forced.

%    --- constants from 1976 std. atmosphere
r     = 1716.55915670803;
gamma = 1.4;
g     = 32.17405;
re    = 20855531.5;
tsl   = 288.15 * 1.8;
psl   = 2116.22;
hsl   = 0.;
sldens = 0.0023769;                 % atmospheric density at sea level
slpr   = 2116.220;                  % sea level pressure, psf

%---------------------------------------------------------------------
%    conversion from metric lapse rate to english lapse rate
%    meters/0.3048 = ft
%    Kelvin * 1.8 = Rankine
rm2ft = 1000.0/0.3048;
conlapse = 1.8/rm2ft;

%  ---- convert geometric alt. to geopotential alt.
h     = (re*z)/(re+z);
 
%  ---- ensure we are in layer one (based on geopotential alt)
if (h > 11*rm2ft) % 11 km
  %fprintf(1,'Error, atmosphere model out of range %f, Limiting...\n',h);
  h=11*rm2ft;
end
if (h<0)
  %fprintf(1,'Error, atmosphere model out of range %f, Limiting...\n',h);
  h=0;
end

a1     = -6.5*conlapse;
t1     = tsl + a1*(h-hsl);
del1   = (t1/tsl)^(-g/r/a1);
p1     = del1 * psl;

%   ---- apply temperature increment from standard day*/
t1     = t1 + dt;

%   ---- calculate density from eqn. of state w/ corrected temp.*/
rho1   = p1 / (r * t1);
 
%   ---- calculate speed of sound w/ corrected temp.*/
c1     = sqrt(gamma * (r * t1));
 

% Calculate outputs
y(1) = rho1;
y(2) = p1;
y(3) = t1 / 1.8; % output temperature  in Kelvin
y(4) = c1;
y(5) = y(2) / slpr;         % pressure ratio
y(6) = sqrt(y(1)/sldens);   % SQUARE ROOT OF DENSITY RATIO

== matlab function gtm_design/GTM_T2/AuxiliaryVariables/Embedded MATLAB Function ==
  data: omega input; euler input; v input; n_body output; v_dot input
function n_body = accels(omega,euler,v,v_dot)
% Compute body-axis accelerometer measurements.  
% Inputs:
%       omega: body-axis angular rates, [p q r], in rad/sec
%       euler: Euler angles, [phi theta psi], in rad
%           v: body-axis velocities, [u v w], ft/sec
%       v_dot: body-axis accelerations, [udot vdot wdot], ft/sec^2
%
%
% Author: Austin Murch (Austin.M.Murch@nasa.gov)
% Created: 2/19/2008

g0    = 32.174;
phi   = euler(1);
theta = euler(2);

n_body = (v_dot + cross(omega,v))/g0 - [-sin(theta); cos(theta)*sin(phi); cos(theta)*cos(phi)];
